simulink model "Mdl_9"  (R2017b)
settings: Solver=VariableStepAuto  StartTime=0.0  StopTime=10.0  RelTol=1e-3
undefined symbols (not defined in the file): A, B, C, D, simSwitch, u0, x0
settings Model: Creator=lasse  LastModifiedBy=lasse
settings DataIOCC: SaveFinalState=on  SaveFormat=StructureWithTime  SaveState=on  SignalLogging=off  DSMLogging=off

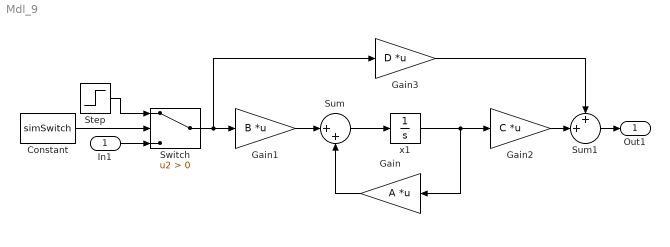
== system Mdl_9 ==
  In1 : Inport  PortDimensions=2
  Constant : Constant  Value=simSwitch
  Gain : Gain  Gain=A  Multiplication=Matrix(K*u)
  Gain1 : Gain  Gain=B  Multiplication=Matrix(K*u)
  Gain2 : Gain  Gain=C  Multiplication=Matrix(K*u)
  Gain3 : Gain  Gain=D  Multiplication=Matrix(K*u)
  Step : Step  After=u0  SampleTime=0
  Sum : Sum  Inputs=|++
  Sum1 : Sum  Inputs=++|
  Switch : Switch  Criteria=u2 > Threshold
  x1 : Integrator  InitialCondition=x0
  Out1 : Outport
  wires:
  x1/1 -> Gain/1, Gain2/1
  Gain1/1 -> Sum/1
  Sum/1 -> x1/1
  Gain/1 -> Sum/2
  Gain2/1 -> Sum1/2
  Gain3/1 -> Sum1/1
  Sum1/1 -> Out1/1
  Step/1 -> Switch/1
  In1/1 -> Switch/3
  Constant/1 -> Switch/2
  Switch/1 -> Gain3/1, Gain1/1
